simulink model "speed_controller"  (R2020b)
settings: Solver=FixedStepDiscrete  StartTime=0.0  StopTime=0.5  FixedStep=double(Ts)  RelTol=1e-3
undefined symbols (not defined in the file): DiscIntNeverNeededParam, FiltFreq, Ki, Kp, trqMax_Nm, Ts
libraries: simulink x1
settings Model: DataDictionary=hvb.sldd  Creator=Dmitry  LastModifiedBy=Dmitry

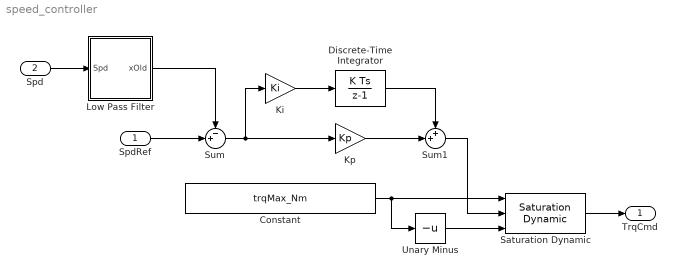
== system speed_controller ==
  SpdRef : Inport  OutDataTypeStr=single  Unit=rpm
      settings: AttributesFormatString=%<Unit>
  Spd : Inport  Port=2  OutDataTypeStr=single  Unit=rpm
      settings: AttributesFormatString=%<Unit>
  Constant : Constant  Value=trqMax_Nm
  Discrete-Time Integrator : DiscreteIntegrator  SampleTime=-1  LimitOutput=on  UpperSaturationLimit=40  LowerSaturationLimit=-40  ICPrevOutput=DiscIntNeverNeededParam  ICPrevScaledInput=DiscIntNeverNeededParam
  Ki : Gain  Gain=Ki
  Kp : Gain  Gain=Kp
  Low Pass Filter : Subsystem
  Saturation Dynamic : simulink/Discontinuities/Saturation Dynamic  OutMin=[]  OutMax=[]  OutDataTypeStr=Inherit: Same as second input  OutDataType=fixdt(1, 16)  OutScaling=2^-10  DoSatur=off
  Sum : Sum  Inputs=-+|
  Sum1 : Sum  Inputs=++|
  Unary Minus : UnaryMinus
  TrqCmd : Outport  OutDataTypeStr=single  Unit=N*m  VectorParamsAs1DForOutWhenUnconnected=off
      settings: AttributesFormatString=%<Unit>
  wires:
  Discrete-Time Integrator/1 -> Sum1/1
  Ki/1 -> Discrete-Time Integrator/1
  SpdRef/1 -> Sum/2
  Kp/1 -> Sum1/2
  Saturation Dynamic/1 -> TrqCmd/1
  Spd/1 -> Low Pass Filter/1(Spd)
  Low Pass Filter/1(xOld) -> Sum/1
  Sum/1 -> Kp/1, Ki/1
  Sum1/1 -> Saturation Dynamic/2
  Unary Minus/1 -> Saturation Dynamic/3
  Constant/1 -> Saturation Dynamic/1, Unary Minus/1

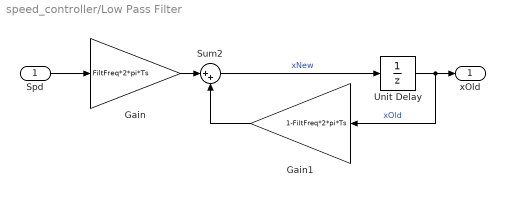
== system speed_controller/Low Pass Filter ==
  Spd : Inport
  Gain : Gain  Gain=FiltFreq*2*pi*Ts
  Gain1 : Gain  Gain=1-FiltFreq*2*pi*Ts
  Sum2 : Sum  Inputs=|++
  Unit Delay : UnitDelay  SampleTime=-1  HasFrameUpgradeWarning=on
  xOld : Outport
  wires:
  Gain1/1 -> Sum2/2
  Gain/1 -> Sum2/1
  Spd/1 -> Gain/1
  Sum2/1 -> Unit Delay/1  "xNew"
  Unit Delay/1 -> Gain1/1, xOld/1  "xOld"
